simulink model "Ej3_v2"  (R2015a)
settings: Solver=ode45  StartTime=0.0  StopTime=9  RelTol=1e-3
libraries: cstblocks x6, simulink x3
settings Model: Creator=Daniel  LastModifiedBy=Daniel

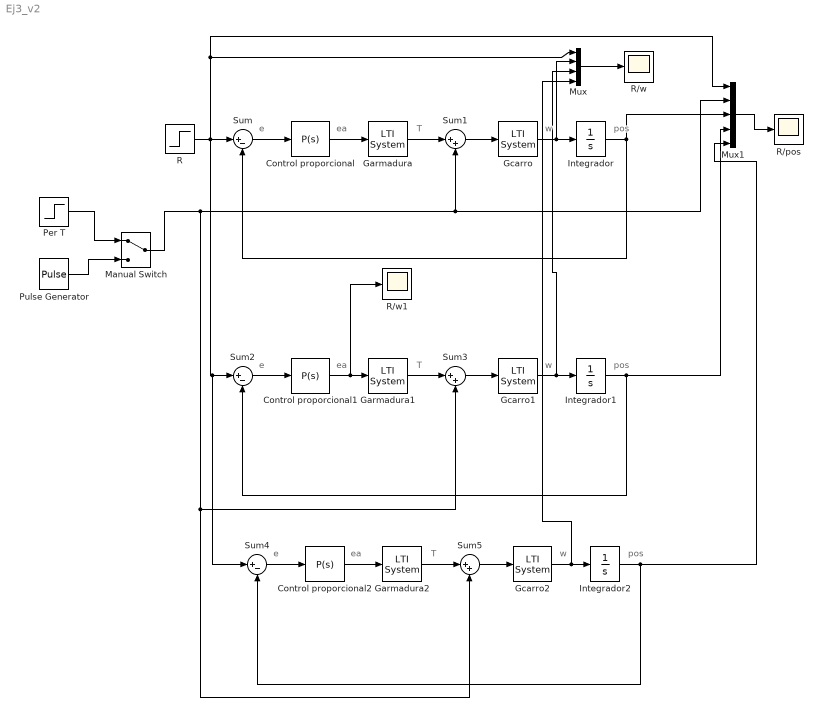
== system Ej3_v2 ==
  note: T
  note: pos
  note: w
  note: e
  note: ea
  note: T
  note: pos
  note: w
  note: e
  note: ea
  note: T
  note: pos
  note: w
  note: e
  note: ea
  Control proporcional : simulink/Continuous/PID Controller  Controller=P  TimeDomain=Continuous-time  SampleTime=-1  IntegratorMethod=Forward Euler  FilterMethod=Forward Euler  Form=Ideal  UseFilter=on  ControllerParametersSource=internal  P=20  I=0  D=0  N=100  InitialConditionSource=internal  InitialConditionForIntegrator=0  InitialConditionForFilter=0  ExternalReset=none  LimitOutput=off  UpperSaturationLimit=12  LowerSaturationLimit=-inf  LinearizeAsGain=on  AntiWindupMode=none  Kb=1  TrackingMode=off  Kt=1  PParamMin=[]  PParamMax=[]  IParamMin=[]  IParamMax=[]  DParamMin=[]  DParamMax=[]  NParamMin=[]  NParamMax=[]  KbParamMin=[]  KbParamMax=[]  KtParamMin=[]  KtParamMax=[]  POutMin=[]  POutMax=[]  IOutMin=[]  IOutMax=[]  DOutMin=[]  DOutMax=[]  NOutMin=[]  NOutMax=[]  KbOutMin=[]  KbOutMax=[]  KtOutMin=[]  KtOutMax=[]  IntegratorOutMin=[]  IntegratorOutMax=[]  FilterOutMin=[]  FilterOutMax=[]  SumOutMin=[]  SumOutMax=[]  SumI1OutMin=[]  SumI1OutMax=[]  SumI2OutMin=[]  SumI2OutMax=[]  SumI3OutMin=[]  SumI3OutMax=[]  SumDOutMin=[]  SumDOutMax=[]  SaturationOutMin=[]  SaturationOutMax=[]  IntegratorContinuousStateAttributes=''  IntegratorStateMustResolveToSignalObject=off  IntegratorRTWStateStorageClass=Auto  FilterContinuousStateAttributes=''  FilterStateMustResolveToSignalObject=off  FilterRTWStateStorageClass=Auto  DifferentiatorICPrevScaledInput=0  DifferentiatorOutMin=[]  DifferentiatorOutMax=[]
  Control proporcional1 : simulink/Continuous/PID Controller  Controller=P  TimeDomain=Continuous-time  SampleTime=-1  IntegratorMethod=Forward Euler  FilterMethod=Forward Euler  Form=Ideal  UseFilter=on  ControllerParametersSource=internal  P=40  I=0  D=0  N=100  InitialConditionSource=internal  InitialConditionForIntegrator=0  InitialConditionForFilter=0  ExternalReset=none  LimitOutput=off  UpperSaturationLimit=12  LowerSaturationLimit=-inf  LinearizeAsGain=on  AntiWindupMode=none  Kb=1  TrackingMode=off  Kt=1  PParamMin=[]  PParamMax=[]  IParamMin=[]  IParamMax=[]  DParamMin=[]  DParamMax=[]  NParamMin=[]  NParamMax=[]  KbParamMin=[]  KbParamMax=[]  KtParamMin=[]  KtParamMax=[]  POutMin=[]  POutMax=[]  IOutMin=[]  IOutMax=[]  DOutMin=[]  DOutMax=[]  NOutMin=[]  NOutMax=[]  KbOutMin=[]  KbOutMax=[]  KtOutMin=[]  KtOutMax=[]  IntegratorOutMin=[]  IntegratorOutMax=[]  FilterOutMin=[]  FilterOutMax=[]  SumOutMin=[]  SumOutMax=[]  SumI1OutMin=[]  SumI1OutMax=[]  SumI2OutMin=[]  SumI2OutMax=[]  SumI3OutMin=[]  SumI3OutMax=[]  SumDOutMin=[]  SumDOutMax=[]  SaturationOutMin=[]  SaturationOutMax=[]  IntegratorContinuousStateAttributes=''  IntegratorStateMustResolveToSignalObject=off  IntegratorRTWStateStorageClass=Auto  FilterContinuousStateAttributes=''  FilterStateMustResolveToSignalObject=off  FilterRTWStateStorageClass=Auto  DifferentiatorICPrevScaledInput=0  DifferentiatorOutMin=[]  DifferentiatorOutMax=[]
  Control proporcional2 : simulink/Continuous/PID Controller  Controller=P  TimeDomain=Continuous-time  SampleTime=-1  IntegratorMethod=Forward Euler  FilterMethod=Forward Euler  Form=Ideal  UseFilter=on  ControllerParametersSource=internal  P=80  I=0  D=0  N=100  InitialConditionSource=internal  InitialConditionForIntegrator=0  InitialConditionForFilter=0  ExternalReset=none  LimitOutput=off  UpperSaturationLimit=12  LowerSaturationLimit=-inf  LinearizeAsGain=on  AntiWindupMode=none  Kb=1  TrackingMode=off  Kt=1  PParamMin=[]  PParamMax=[]  IParamMin=[]  IParamMax=[]  DParamMin=[]  DParamMax=[]  NParamMin=[]  NParamMax=[]  KbParamMin=[]  KbParamMax=[]  KtParamMin=[]  KtParamMax=[]  POutMin=[]  POutMax=[]  IOutMin=[]  IOutMax=[]  DOutMin=[]  DOutMax=[]  NOutMin=[]  NOutMax=[]  KbOutMin=[]  KbOutMax=[]  KtOutMin=[]  KtOutMax=[]  IntegratorOutMin=[]  IntegratorOutMax=[]  FilterOutMin=[]  FilterOutMax=[]  SumOutMin=[]  SumOutMax=[]  SumI1OutMin=[]  SumI1OutMax=[]  SumI2OutMin=[]  SumI2OutMax=[]  SumI3OutMin=[]  SumI3OutMax=[]  SumDOutMin=[]  SumDOutMax=[]  SaturationOutMin=[]  SaturationOutMax=[]  IntegratorContinuousStateAttributes=''  IntegratorStateMustResolveToSignalObject=off  IntegratorRTWStateStorageClass=Auto  FilterContinuousStateAttributes=''  FilterStateMustResolveToSignalObject=off  FilterRTWStateStorageClass=Auto  DifferentiatorICPrevScaledInput=0  DifferentiatorOutMin=[]  DifferentiatorOutMax=[]
  Garmadura : cstblocks/LTI System  sys=Garm  IC=[]
  Garmadura1 : cstblocks/LTI System  sys=Garm  IC=[]
  Garmadura2 : cstblocks/LTI System  sys=Garm  IC=[]
  Gcarro : cstblocks/LTI System  sys=Gcar  IC=[]
  Gcarro1 : cstblocks/LTI System  sys=Gcar  IC=[]
  Gcarro2 : cstblocks/LTI System  sys=Gcar  IC=[]
  Integrador : Integrator
  Integrador1 : Integrator
  Integrador2 : Integrator
  Manual Switch : ManualSwitch
  Mux : Mux
  Mux1 : Mux  Inputs=5
  Per T : Step  Time=1.5  SampleTime=0
  Pulse Generator : DiscretePulseGenerator  PulseType=Time based  Period=0.2  PulseWidth=50
  R : Step  Time=0  After=0.6  SampleTime=0
  R/pos : Scope
      settings: SaveName=pos
  R/w : Scope
      settings: YMin=0  YMax=0.6  SaveName=w
  R/w1 : Scope
      settings: YMin=0  YMax=0.6  SaveName=w1
  Sum : Sum  Inputs=|+-
  Sum1 : Sum  Inputs=|++
  Sum2 : Sum  Inputs=|+-
  Sum3 : Sum  Inputs=|++
  Sum4 : Sum  Inputs=|+-
  Sum5 : Sum  Inputs=|++
  wires:
  Sum/1 -> Control proporcional/1
  Control proporcional/1 -> Garmadura/1
  Gcarro/1 -> Mux/2, Integrador/1
  Mux1/1 -> R/pos/1
  Mux/1 -> R/w/1
  Integrador/1 -> Mux1/3, Sum/2
  Garmadura/1 -> Sum1/1
  Sum1/1 -> Gcarro/1
  Sum2/1 -> Control proporcional1/1
  Control proporcional1/1 -> R/w1/1, Garmadura1/1
  Gcarro1/1 -> Mux/3, Integrador1/1
  Integrador1/1 -> Mux1/4, Sum2/2
  Garmadura1/1 -> Sum3/1
  Sum3/1 -> Gcarro1/1
  Sum4/1 -> Control proporcional2/1
  Control proporcional2/1 -> Garmadura2/1
  Gcarro2/1 -> Mux/4, Integrador2/1
  R/1 -> Sum4/1, Sum2/1, Mux/1, Mux1/1, Sum/1
  Integrador2/1 -> Mux1/5, Sum4/2
  Garmadura2/1 -> Sum5/1
  Sum5/1 -> Gcarro2/1
  Manual Switch/1 -> Sum5/2, Sum3/2, Mux1/2, Sum1/2
  Pulse Generator/1 -> Manual Switch/2
  Per T/1 -> Manual Switch/1
